simulink model "sampleModel1772_5_sub_sub_sub"  (R2023a)
settings: Solver=VariableStepAuto  StartTime=0.0  StopTime=10.0  RelTol=1e-3
libraries: hdlsllib x1, simulink x1
settings Model: Creator=user1  LastModifiedBy=user1

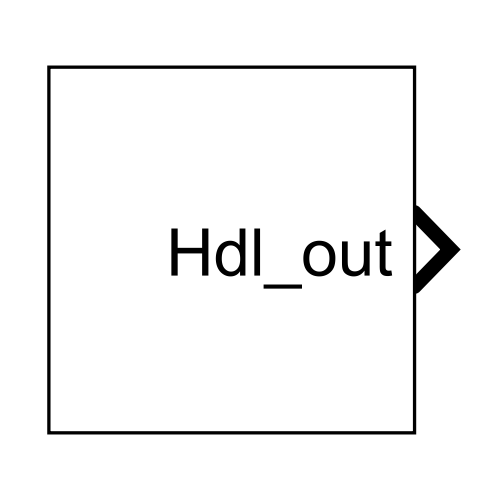
[thumbnail: Simulink's stored preview of the top-level diagram]
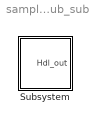
== system sampleModel1772_5_sub_sub_sub ==
  Subsystem : Subsystem

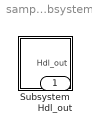
== system sampleModel1772_5_sub_sub_sub/Subsystem ==
  Subsystem : Subsystem
  Hdl_out : Outport  OutDataTypeStr=uint8

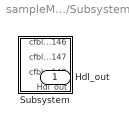
== system sampleModel1772_5_sub_sub_sub/Subsystem/Subsystem ==
  Subsystem : Subsystem
  Hdl_out : Outport  OutDataTypeStr=uint8

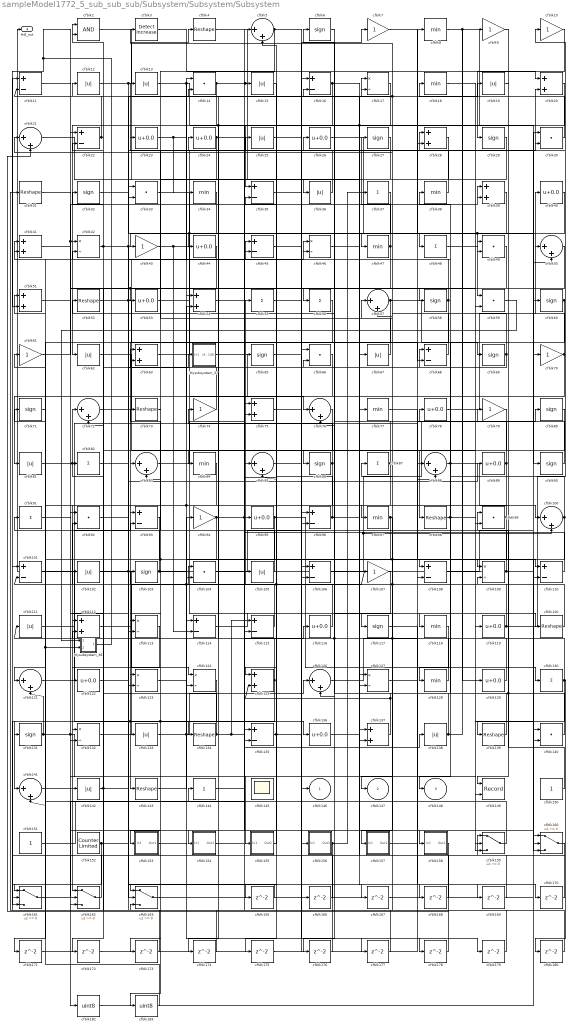
== system sampleModel1772_5_sub_sub_sub/Subsystem/Subsystem/Subsystem ==
  Mysubsystem_36 : Subsystem  TreatAsAtomicUnit=on  RTWFcnName=Mysubsystem_36
      settings: RTWFcnNameOpts=User specified  RTWFileNameOpts=Use function name
  Mysubsystem_37 : Subsystem  TreatAsAtomicUnit=on  RTWFcnName=Mysubsystem_37
      settings: RTWFcnNameOpts=User specified  RTWFileNameOpts=Use function name
  cfblk{7,9..10,43,61,70,74,79,94,107} (10 alike) : Gain  OutDataTypeStr=uint8
  cfblk{5,21,50,57,72,76,83,85,88,100,121,126,141} (13 alike) : Sum  Inputs=|++  OutDataTypeStr=uint8
  cfblk{11,16,22,35,45,68,93,96,101,106,108,110,114..115,135} (15 alike) : Sum  Inputs=+-  OutDataTypeStr=uint8
  cfblk{12..13,15,19,25,36,62,67,81,102,105,111,133,138,142} (15 alike) : Abs  OutDataTypeStr=uint8  SaturateOnIntegerOverflow=off
  cfblk{6,27,29,32,58,60,65,69,71,80,86,90,103,117,131} (15 alike) : Signum
  cfblk{14,30,33,49,59,66,92,99,104,140} (10 alike) : DotProduct  OutDataTypeStr=uint8
  cfblk{17,42,46,109,113,123..124,127,132} (9 alike) : Product  Inputs=*/  OutDataTypeStr=uint8  RndMeth=Zero  SaturateOnIntegerOverflow=on
  cfblk{20,28,39,41,51,54,63,75,112,125,137} (11 alike) : Sum  OutDataTypeStr=uint8
  cfblk{23..24,26,40,44,53,78,89,95,116,119,122,129,136} (14 alike) : Bias  Bias=0.0  SaturateOnIntegerOverflow=off
  cfblk{8,18,34,38,47,77,84,97,118,128} (10 alike) : MinMax  OutDataTypeStr=uint8
  cfblk{4,31,52,73,98,120,134,139,143} (9 alike) : Reshape
  cfblk{37,48,55..56,82,87,91,130,144} (9 alike) : Sum  Inputs=+  OutDataTypeStr=uint8
  cfblk145 : Scope
      settings: Floating=on
  cfblk149 : Record  FileSettingsInternal="{\"entries\":[{\"content\":{\"excelSettings\":{\"content\":{},\"type\":\"Streamout.ExcelSettings\"}},\"type\":\"Streamout.FileSettingStorage\",\"uuid\":\"\"}],\"packageUris\":[\"http:\\/\\/schema.mathworks.com\\/mf0\\/streamout_blocks\\/R2020a\"],\"version\":\"1.0\"}"  Layout=[1 1]  SignalsInternal="{\"entries\":[{\"content\":{\"signals\":[{\"content\":{\"blockPath\":[],\"dimensions\":[1],\"domain\":\"\",\"lineColor\":\"#a2142f\",\"plots\":[1],\"port\":1,\"signalID\":40516,\"signalName\":\"cfblk9\"},\"type\":\"RecordBlkView.Signal\",\"uuid\":\"\"},{\"content\":{\"blockPath\":[],\"dimensions\":[1],\"domain\":\"\",\"lineColor\":\"#139fff\",\"plots\":[1],\"port\":2,\"signalID\":40519,\"signalName\":\"cfblk131\"},\"type\":\"RecordBlkView.Signal\",\"uuid\":\"\"}]},\"type\":\"RecordBlkView.InputSignals\",\"uuid\":\"\"}],\"packageUris\":[\"http:\\/\\/schema.mathworks.com\\/mf0\\/streamout_blocks\\/R2020a\"],\"version\":\"1.0\"}"  VisualizationBindings="{\"xyplotplugin\":{\"info\":[{\"series\":[{\"bindingParametersList\":[{\"parameter\":\"X-Axis\",\"signalID\":40516,\"signalName\":\"cfblk9\"},{\"parameter\":\"Y-Axis\",\"signalID\":40519,\"signalName\":\"cfblk131\"}],\"seriesID\":48563}],\"subplotID\":1}]}}"  CompatibilityTag=XY  st=-1
  cfblk150 : Constant  OutDataTypeStr=uint8  SampleTime=-1
  cfblk151 : Constant  OutDataTypeStr=uint8  SampleTime=-1
  cfblk152 : hdlsllib/Sources/Counter Limited  uplimit=7  tsamp=-1
  cfblk153 : Subsystem
      settings: LibrarySourceBlock=|
      | hdlsllib/Ports &
      | Subsystems/Subsystem
  cfblk154 : Subsystem
      settings: LibrarySourceBlock=|
      | hdlsllib/Ports &
      | Subsystems/Subsystem
  cfblk155 : Subsystem
      settings: LibrarySourceBlock=|
      | hdlsllib/Ports &
      | Subsystems/Subsystem
  cfblk156 : Subsystem
      settings: LibrarySourceBlock=|
      | hdlsllib/Ports &
      | Subsystems/Subsystem
  cfblk157 : Subsystem
      settings: LibrarySourceBlock=|
      | hdlsllib/Ports &
      | Subsystems/Subsystem
  cfblk158 : Subsystem
      settings: LibrarySourceBlock=|
      | hdlsllib/Ports &
      | Subsystems/Subsystem
  cfblk{159..163} (5 alike) : Switch  OutDataTypeStr=uint8  SaturateOnIntegerOverflow=off  InputSameDT=off
  cfblk{165..180} (16 alike) : Delay  SampleTime=1
  cfblk182 : DataTypeConversion  OutDataTypeStr=uint8  SaturateOnIntegerOverflow=off  RndMeth=Floor
  cfblk183 : DataTypeConversion  OutDataTypeStr=uint8  SaturateOnIntegerOverflow=off  RndMeth=Floor
  cfblk2 : Logic  AllPortsSameDT=off  OutDataTypeStr=boolean
  cfblk3 : simulink/Logic and Bit Operations/Detect Increase  vinit=0.0  OutDataTypeStr=uint8
      settings: LibrarySourceBlock=|
      | hdlsllib/Logic and Bit
      | Operations/Detect
      | Increase
  cfblk146 : Outport  OutDataTypeStr=uint8  VectorParamsAs1DForOutWhenUnconnected=off
  cfblk147 : Outport  Port=2  OutDataTypeStr=uint8  VectorParamsAs1DForOutWhenUnconnected=off
  cfblk148 : Outport  Port=3  OutDataTypeStr=uint8  VectorParamsAs1DForOutWhenUnconnected=off
  Hdl_out : Outport  Port=4  OutDataTypeStr=uint8
  wires:
  cfblk80/1 -> cfblk143/1
  cfblk102/1 -> cfblk160/2, cfblk124/1
  cfblk118/1 -> cfblk128/1
  cfblk14/1 -> cfblk62/1, cfblk15/1, cfblk70/1
  cfblk70/1 -> cfblk75/2, cfblk40/1
  cfblk140/1 -> cfblk109/2, cfblk103/1
  cfblk159/1 -> cfblk41/1
  cfblk142/1 -> cfblk169/1, cfblk112/2
  cfblk43/1 -> cfblk114/2, cfblk47/1
  cfblk119/1 -> cfblk28/1, cfblk17/2, cfblk85/1
  cfblk132/1 -> cfblk55/1
  cfblk5/1 -> cfblk158/1(In1), cfblk93/1
  cfblk53/1 -> cfblk76/1
  cfblk12/1 -> cfblk48/1, cfblk4/1
  cfblk60/1 -> cfblk148/1, cfblk10/1
  cfblk87/1 -> cfblk63/1, cfblk162/1
  cfblk39/1 -> cfblk126/2, cfblk59/1
  cfblk139/1 -> cfblk78/1
  cfblk20/1 -> cfblk35/1
  cfblk4/1 -> cfblk36/1
  cfblk34/1 -> cfblk113/1
  cfblk32/1 -> cfblk24/1
  cfblk112/1 -> cfblk124/2
  cfblk79/1 -> cfblk98/1
  cfblk10/1 -> cfblk29/1
  cfblk95/1 -> cfblk130/1, cfblk183/1, cfblk123/2
  cfblk155/1(Out1) -> cfblk35/2
  cfblk28/1 -> cfblk43/1
  cfblk81/1 -> cfblk54/2, cfblk72/1
  cfblk77/1 -> cfblk110/1
  cfblk161/1 -> cfblk144/1
  cfblk121/1 -> cfblk28/2
  cfblk72/1 -> cfblk14/1
  cfblk130/1 -> cfblk180/1, cfblk159/3, cfblk105/1
  cfblk78/1 -> cfblk50/1
  cfblk65/1 -> cfblk156/1(In1)
  cfblk2/1 -> cfblk77/1
  cfblk110/1 -> cfblk95/1
  cfblk22/1 -> cfblk2/1, cfblk12/1
  cfblk51/1 -> cfblk142/1
  cfblk75/1 -> cfblk117/1
  cfblk24/1 -> cfblk110/2, cfblk163/1
  cfblk96/1 -> cfblk19/1, cfblk45/1
  cfblk156/1(Out1) -> cfblk37/1, cfblk31/1
  cfblk58/1 -> cfblk6/1, cfblk83/1
  cfblk109/1 -> Hdl_out/1, cfblk5/2, cfblk160/1
  cfblk19/1 -> cfblk139/1
  cfblk3/1 -> cfblk20/1
  cfblk115/1 -> cfblk51/1
  cfblk98/1 -> cfblk140/2, cfblk68/1
  cfblk54/1 -> cfblk26/1
  cfblk74/1 -> cfblk32/1
  cfblk89/1 -> cfblk52/1, cfblk162/2
  cfblk100/1 -> cfblk102/1, cfblk41/2
  cfblk9/1 -> cfblk149/1
  cfblk111/1 -> cfblk93/2
  cfblk136/1 -> cfblk67/1
  cfblk45/1 -> cfblk106/1
  cfblk30/1 -> cfblk18/1
  cfblk55/1 -> cfblk96/2
  cfblk93/1 -> cfblk121/1
  cfblk113/1 -> cfblk132/1
  cfblk50/1 -> cfblk53/1, cfblk162/3
  cfblk68/1 -> cfblk21/1
  cfblk134/1 -> cfblk82/1, cfblk115/1, cfblk116/1
  cfblk25/1 -> cfblk7/1
  cfblk8/1 -> cfblk129/1, cfblk90/1
  cfblk49/1 -> cfblk86/1
  cfblk71/1 -> cfblk161/1
  cfblk99/1 -> cfblk97/1, cfblk172/1, cfblk157/1(In1)
  cfblk131/1 -> cfblk121/2, cfblk149/2, cfblk155/1(In1)
  cfblk66/1 -> cfblk81/1
  cfblk120/1 -> cfblk65/1, cfblk101/2
  cfblk46/1 -> cfblk108/1
  cfblk35/1 -> cfblk59/2
  cfblk157/1(Out1) -> cfblk108/2
  cfblk150/1 -> cfblk99/1
  cfblk101/1 -> cfblk136/1
  cfblk26/1 -> cfblk60/1
  cfblk163/1 -> cfblk8/1
  cfblk38/1 -> cfblk13/1
  cfblk18/1 -> cfblk119/1
  cfblk69/1 -> cfblk63/2, cfblk11/2, cfblk3/1
  cfblk127/1 -> cfblk80/1
  cfblk162/1 -> cfblk71/1
  cfblk33/1 -> cfblk137/1, cfblk120/1
  cfblk52/1 -> cfblk30/2, cfblk68/2
  cfblk114/1 -> cfblk118/1
  cfblk11/1 -> cfblk58/1, cfblk42/1
  cfblk141/1 -> cfblk154/1(In1)
  cfblk56/1 -> Mysubsystem_36/2(In2), cfblk141/2
  cfblk133/1 -> cfblk178/1, cfblk126/1
  cfblk41/1 -> cfblk92/1
  cfblk116/1 -> cfblk92/2
  cfblk152/1 -> cfblk89/1, cfblk161/2
  cfblk97/1 -> cfblk173/1, cfblk147/1
  cfblk37/1 -> cfblk123/1
  cfblk31/1 -> cfblk113/2
  cfblk135/1 -> cfblk85/2, cfblk39/1
  cfblk90/1 -> cfblk57/2
  cfblk137/1 -> cfblk125/2, cfblk46/2, cfblk111/1
  cfblk63/1 -> cfblk20/2
  cfblk154/1(Out1) -> cfblk138/1
  cfblk36/1 -> cfblk25/1
  cfblk7/1 -> cfblk49/1
  cfblk128/1 -> cfblk66/2, cfblk87/1
  cfblk86/1 -> cfblk132/2, cfblk74/1
  cfblk6/1 -> cfblk56/1
  cfblk108/1 -> cfblk50/2
  cfblk138/1 -> cfblk9/1, cfblk76/2
  cfblk62/1 -> cfblk99/2
  cfblk143/1 -> cfblk107/1, cfblk94/1
  cfblk17/1 -> cfblk137/2, cfblk44/1, cfblk33/2
  cfblk47/1 -> cfblk27/1, cfblk134/1
  cfblk158/1(Out1) -> cfblk21/2
  cfblk105/1 -> cfblk73/1
  cfblk124/1 -> cfblk141/1
  cfblk44/1 -> cfblk112/1
  cfblk103/1 -> cfblk109/1, cfblk61/1
  cfblk48/1 -> cfblk49/2
  cfblk123/1 -> cfblk114/1
  cfblk67/1 -> cfblk23/1
  cfblk83/1 -> cfblk45/2
  cfblk104/1 -> cfblk16/1
  cfblk73/1 -> cfblk83/2
  cfblk94/1 -> cfblk131/1, cfblk160/3, cfblk16/2
  cfblk88/1 -> cfblk38/1, cfblk100/1
  cfblk106/1 -> cfblk100/2, cfblk79/1
  cfblk125/1 -> cfblk14/2, cfblk153/1(In1), cfblk133/1, cfblk161/3
  cfblk76/1 -> cfblk122/1
  cfblk61/1 -> cfblk39/2
  cfblk151/1 -> cfblk5/1
  cfblk160/1 -> cfblk159/1
  cfblk57/1 -> cfblk125/1, cfblk69/1
  cfblk129/1 -> cfblk104/1
  cfblk84/1 -> cfblk171/1, cfblk104/2
  cfblk27/1 -> cfblk84/1
  cfblk144/1 -> cfblk75/1
  cfblk126/1 -> cfblk88/1
  cfblk23/1 -> cfblk34/1, cfblk54/1
  cfblk16/1 -> cfblk168/1, cfblk115/2
  cfblk42/1 -> cfblk2/2, cfblk135/2, cfblk17/1
  cfblk82/1 -> cfblk46/1
  cfblk13/1 -> cfblk159/2, cfblk127/2
  cfblk29/1 -> cfblk165/1
  cfblk165/1 -> cfblk163/2
  cfblk21/1 -> cfblk166/1
  cfblk166/1 -> cfblk22/2
  cfblk92/1 -> cfblk167/1
  cfblk167/1 -> cfblk140/1
  cfblk168/1 -> cfblk127/1
  cfblk169/1 -> cfblk96/1
  cfblk117/1 -> cfblk170/1
  cfblk170/1 -> cfblk101/1
  cfblk171/1 -> cfblk88/2
  cfblk172/1 -> cfblk106/2
  cfblk173/1 -> cfblk72/2
  cfblk40/1 -> cfblk174/1
  cfblk174/1 -> cfblk42/2
  cfblk15/1 -> cfblk175/1
  cfblk175/1 -> cfblk66/1
  cfblk107/1 -> cfblk176/1
  cfblk176/1 -> cfblk163/3
  cfblk153/1(Out1) -> cfblk177/1
  cfblk177/1 -> cfblk33/1
  cfblk178/1 -> cfblk11/1
  cfblk85/1 -> cfblk179/1
  cfblk179/1 -> cfblk135/1
  cfblk180/1 -> cfblk57/1
  cfblk91/1 -> cfblk182/1
  cfblk182/1 -> cfblk30/1
  cfblk183/1 -> cfblk91/1
  Mysubsystem_36/1(Out1) -> cfblk51/2, cfblk22/1
  cfblk59/1 -> Mysubsystem_36/1(In1)
  cfblk122/1 -> Mysubsystem_37/1(In1)
  Mysubsystem_37/1(cfblk146) -> cfblk146/1

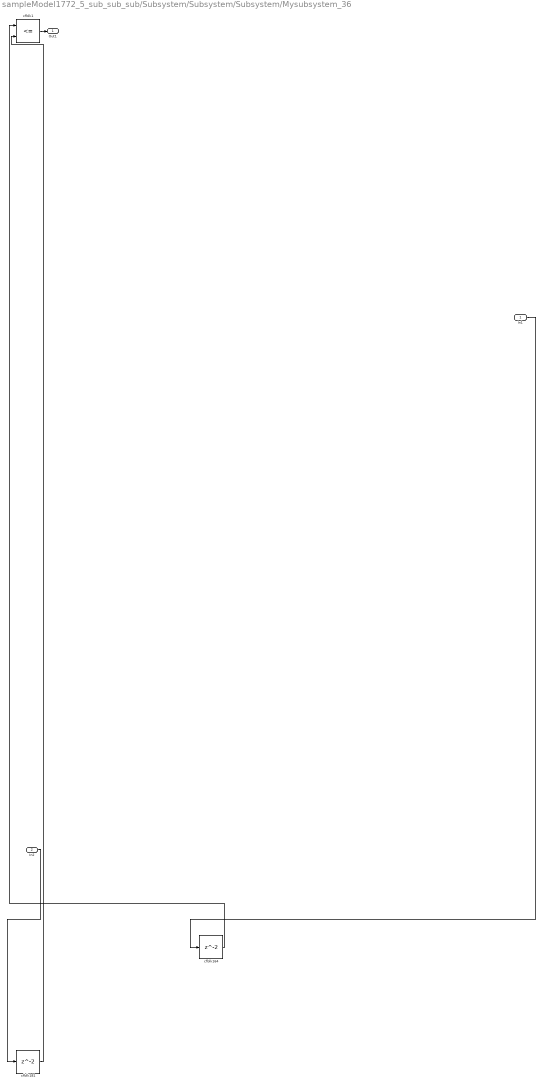
== system sampleModel1772_5_sub_sub_sub/Subsystem/Subsystem/Subsystem/Mysubsystem_36 ==
  In1 : Inport
  In2 : Inport  Port=2
  cfblk1 : RelationalOperator  Operator=<=  OutDataTypeStr=boolean  InputSameDT=off
  cfblk164 : Delay  SampleTime=1
  cfblk181 : Delay  SampleTime=1
  Out1 : Outport
  wires:
  In1/1 -> cfblk164/1
  In2/1 -> cfblk181/1
  cfblk1/1 -> Out1/1
  cfblk181/1 -> cfblk1/2
  cfblk164/1 -> cfblk1/1

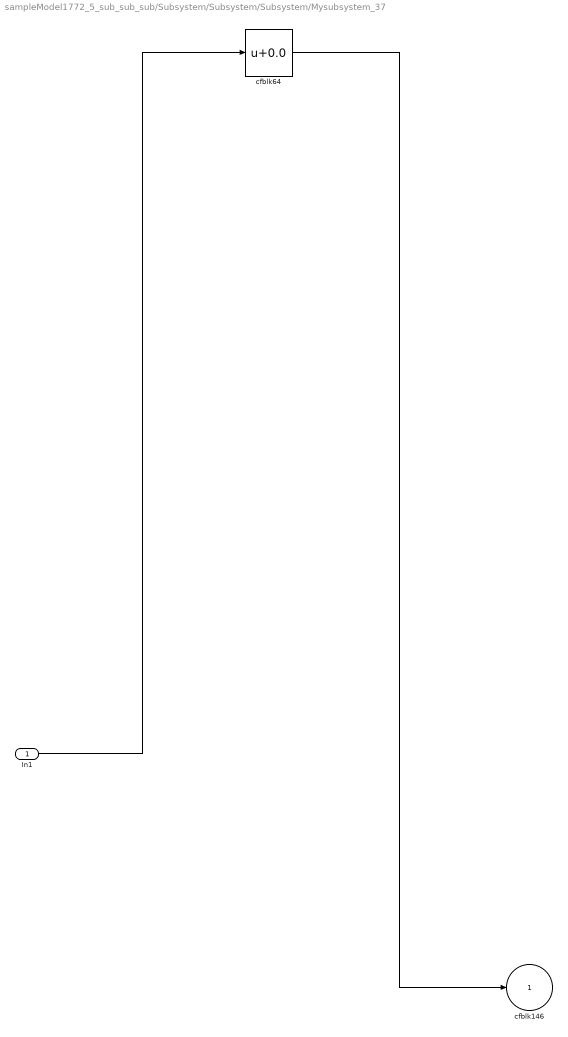
== system sampleModel1772_5_sub_sub_sub/Subsystem/Subsystem/Subsystem/Mysubsystem_37 ==
  In1 : Inport
  cfblk64 : Bias  Bias=0.0  SaturateOnIntegerOverflow=off
  cfblk146 : Outport  VectorParamsAs1DForOutWhenUnconnected=off
  wires:
  In1/1 -> cfblk64/1
  cfblk64/1 -> cfblk146/1

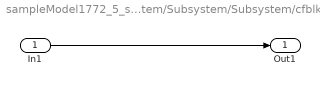
== system sampleModel1772_5_sub_sub_sub/Subsystem/Subsystem/Subsystem/cfblk153 ==
  In1 : Inport
  Out1 : Outport
  wires:
  In1/1 -> Out1/1

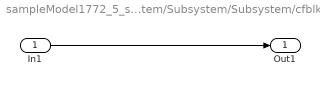
== system sampleModel1772_5_sub_sub_sub/Subsystem/Subsystem/Subsystem/cfblk154 ==
  In1 : Inport
  Out1 : Outport
  wires:
  In1/1 -> Out1/1

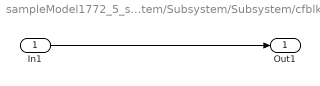
== system sampleModel1772_5_sub_sub_sub/Subsystem/Subsystem/Subsystem/cfblk155 ==
  In1 : Inport
  Out1 : Outport
  wires:
  In1/1 -> Out1/1

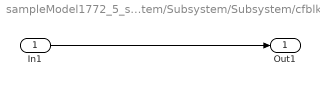
== system sampleModel1772_5_sub_sub_sub/Subsystem/Subsystem/Subsystem/cfblk156 ==
  In1 : Inport
  Out1 : Outport
  wires:
  In1/1 -> Out1/1

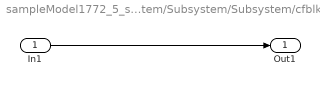
== system sampleModel1772_5_sub_sub_sub/Subsystem/Subsystem/Subsystem/cfblk157 ==
  In1 : Inport
  Out1 : Outport
  wires:
  In1/1 -> Out1/1

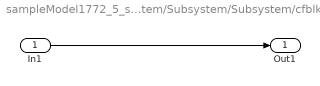
== system sampleModel1772_5_sub_sub_sub/Subsystem/Subsystem/Subsystem/cfblk158 ==
  In1 : Inport
  Out1 : Outport
  wires:
  In1/1 -> Out1/1
